simulink model "Robot"  (R2022a)
settings: Solver=VariableStepAuto  StartTime=0.0  StopTime=10.0  RelTol=1e-3
libraries: robotmaniplib x1
settings Model: Creator=kaspe  LastModifiedBy=kaspe

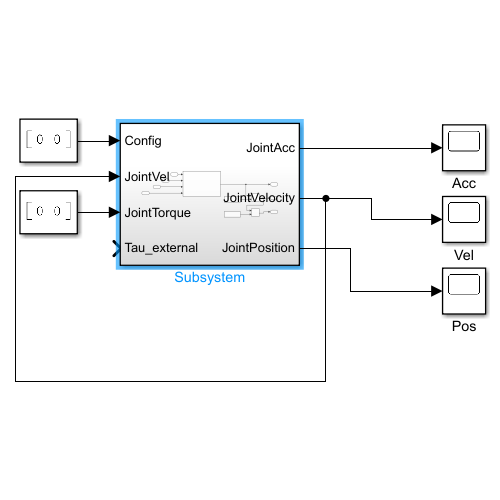
[thumbnail: Simulink's stored preview of the top-level diagram]
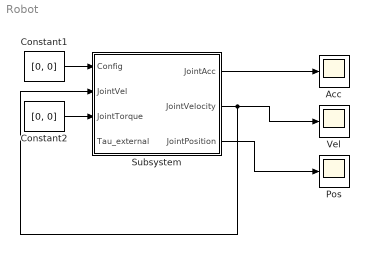
== system Robot ==
  Acc : Scope
  Constant1 : Constant  Value=[0, 0]
  Constant2 : Constant  Value=[0, 0]
  Pos : Scope
  Subsystem : Subsystem
  Vel : Scope
  wires:
  Constant2/1 -> Subsystem/3(JointTorque)
  Subsystem/1(JointAcc) -> Acc/1
  Constant1/1 -> Subsystem/1(Config)
  Subsystem/2(JointVelocity) -> Vel/1, Subsystem/2(JointVel)
  Subsystem/3(JointPosition) -> Pos/1

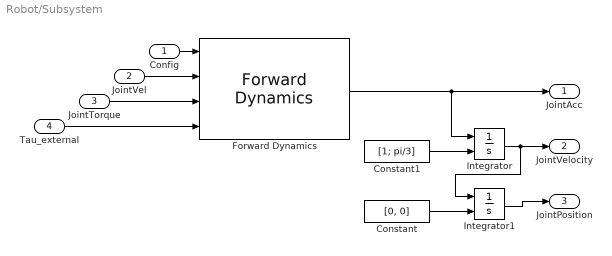
== system Robot/Subsystem ==
  Config : Inport
  JointVel : Inport  Port=2
  JointTorque : Inport  Port=3
  Tau_external : Inport  Port=4
  Constant : Constant  Value=[0, 0]
  Constant1 : Constant  Value=[1; pi/3]
  Forward Dynamics : robotmaniplib/Forward Dynamics  RigidBodyTree=robot  SimulateUsing=Interpreted execution
  Integrator : Integrator  InitialConditionSource=external
  Integrator1 : Integrator  InitialConditionSource=external
  JointAcc : Outport
  JointVelocity : Outport  Port=2
  JointPosition : Outport  Port=3
  wires:
  Integrator/1 -> Integrator1/1, JointVelocity/1
  Integrator1/1 -> JointPosition/1
  Constant1/1 -> Integrator/2
  Constant/1 -> Integrator1/2
  Forward Dynamics/1 -> Integrator/1, JointAcc/1
  JointTorque/1 -> Forward Dynamics/3
  JointVel/1 -> Forward Dynamics/2
  Config/1 -> Forward Dynamics/1
  Tau_external/1 -> Forward Dynamics/4
